simulink model "PhysicalLeanBroth"  (R2026a)
settings: Solver=VariableStepAuto  StopTime=14400
undefined symbols (not defined in the file): Fault_T_Kettle1, Fault_T_Kettle2, Fault_T_Pack, Fault_T_Prep, Fault_T_QC, LB_PackRate_bph, LB_QCRate_bph, LB_Resupply_bph, Recipe_Block_s, Recipe_Count, Resupply_Cutoff_T, Transport_Latency_s, Transport_Rate_bph
(part 2 of 2)

== system PhysicalLeanBroth/PlantServices/ServicesController ==
  in_directive : Inport  PortName=directive
  in_statusTransport : Inport  Port=2  PortName=statusTransport  Element=power_kW
  statusTransportHlth : Inport  Port=2  PortName=statusTransport  Element=health
  in_statusPower : Inport  Port=3  PortName=statusPower  Element=power_kW
  statusPowerHlth : Inport  Port=3  PortName=statusPower  Element=health
  BayHealth : MinMax  Inputs=2
  BayPower : Sum
  HealthPad : Constant
  MemberHealth : Mux
  bayDirective_c1 : Constant  Value=0
  bayDirective_c2 : Constant  Value=0
  bayDirective_c3 : Constant
  bayStatus_c1 : Constant
  bayStatus_c2 : Constant
  bayStatus_c3 : Constant  Value=0
  out_bayDirective : Outport  PortName=bayDirective  Element=cmdType
  bayDirective_el2 : Outport  PortName=bayDirective  Element=targetId
  bayDirective_el3 : Outport  PortName=bayDirective  Element=setpoint
  out_bayStatus : Outport  Port=2  PortName=bayStatus  Element=unitId
  bayStatus_el2 : Outport  Port=2  PortName=bayStatus  Element=opState
  bayStatus_el3 : Outport  Port=2  PortName=bayStatus  Element=faultCode
  bayStatus_el4 : Outport  Port=2  PortName=bayStatus  Element=power_kW
  bayStatus_el5 : Outport  Port=2  PortName=bayStatus  Element=health
  bayStatus_el6 : Outport  Port=2  PortName=bayStatus  Element=lineHealth
  wires:
  BayHealth/1 -> bayStatus_el5/1
  bayStatus_c2/1 -> bayStatus_el2/1
  bayDirective_c3/1 -> bayDirective_el3/1
  statusPowerHlth/1 -> MemberHealth/1, BayHealth/1
  bayStatus_c1/1 -> out_bayStatus/1
  bayDirective_c1/1 -> out_bayDirective/1
  bayStatus_c3/1 -> bayStatus_el3/1
  in_statusTransport/1 -> BayPower/2
  in_statusPower/1 -> BayPower/1
  HealthPad/1 -> MemberHealth/3, MemberHealth/4
  statusTransportHlth/1 -> BayHealth/2, MemberHealth/2
  bayDirective_c2/1 -> bayDirective_el2/1
  BayPower/1 -> bayStatus_el4/1
  MemberHealth/1 -> bayStatus_el6/1

== system PhysicalLeanBroth/ProductionLine/BatchKettle1 ==
  in_preppedBatch : Inport  PortName=preppedBatch  Element=flow_bps
  in_directive : Inport  Port=2  PortName=directive  Element=setpoint
  En_Gate_Fault_T_Kettle1 : Product
  Gate_Fault_T_Kettle1 : Step  Time=Fault_T_Kettle1  InitialValue=1  FinalValue=0  SampleTime=0
  HalfShare : Gain  Gain=0.5
  StateDbl : DataTypeConversion  OutDataTypeStr=double  SaturateOnIntegerOverflow=off  RndMeth=Floor
  ToLitres : Gain  Gain=1800
  Trm22 : Terminator
  Vat : ModelReference  ModelNameDialog=BehCookVat  UsingDefaultArgumentValue=0,0,0,0,0,0,0,0  SimulationMode=Normal  ModelReferenceVersion=1.9
  cookedSoup1_c1 : Constant  Value=0
  cookedSoup1_c2 : Constant  Value=0
  statusCook1_c1 : Constant
  statusCook1_c2 : Constant  Value=0
  out_cookedSoup1 : Outport  PortName=cookedSoup1  Element=batchId
  cookedSoup1_el2 : Outport  PortName=cookedSoup1  Element=volume_L
  cookedSoup1_el3 : Outport  PortName=cookedSoup1  Element=temp_C
  cookedSoup1_el4 : Outport  PortName=cookedSoup1  Element=contamination_ppm
  cookedSoup1_el5 : Outport  PortName=cookedSoup1  Element=flow_bps
  out_statusCook1 : Outport  Port=2  PortName=statusCook1  Element=unitId
  statusCook1_el2 : Outport  Port=2  PortName=statusCook1  Element=opState
  statusCook1_el3 : Outport  Port=2  PortName=statusCook1  Element=faultCode
  statusCook1_el4 : Outport  Port=2  PortName=statusCook1  Element=power_kW
  statusCook1_el5 : Outport  Port=2  PortName=statusCook1  Element=health
  wires:
  statusCook1_c2/1 -> statusCook1_el3/1
  cookedSoup1_c2/1 -> cookedSoup1_el4/1
  in_preppedBatch/1 -> HalfShare/1
  Gate_Fault_T_Kettle1/1 -> statusCook1_el5/1, En_Gate_Fault_T_Kettle1/2
  ToLitres/1 -> cookedSoup1_el2/1
  Vat/3 -> cookedSoup1_el3/1
  statusCook1_c1/1 -> out_statusCook1/1
  Vat/1 -> cookedSoup1_el5/1, ToLitres/1
  in_directive/1 -> En_Gate_Fault_T_Kettle1/1
  cookedSoup1_c1/1 -> out_cookedSoup1/1
  HalfShare/1 -> Vat/1
  En_Gate_Fault_T_Kettle1/1 -> Vat/2
  Vat/2 -> statusCook1_el4/1
  Vat/4 -> StateDbl/1
  Vat/5 -> Trm22/1
  StateDbl/1 -> statusCook1_el2/1

== system PhysicalLeanBroth/ProductionLine/BatchKettle2 ==
  in_preppedBatch : Inport  PortName=preppedBatch  Element=flow_bps
  in_directive : Inport  Port=2  PortName=directive  Element=setpoint
  En_Gate_Fault_T_Kettle2 : Product
  Gate_Fault_T_Kettle2 : Step  Time=Fault_T_Kettle2  InitialValue=1  FinalValue=0  SampleTime=0
  HalfShare : Gain  Gain=0.5
  StateDbl : DataTypeConversion  OutDataTypeStr=double  SaturateOnIntegerOverflow=off  RndMeth=Floor
  ToLitres : Gain  Gain=1800
  Trm23 : Terminator
  Vat : ModelReference  ModelNameDialog=BehCookVat  UsingDefaultArgumentValue=0,0,0,0,0,0,0,0  SimulationMode=Normal  ModelReferenceVersion=1.9
  cookedSoup2_c1 : Constant  Value=0
  cookedSoup2_c2 : Constant  Value=0
  statusCook2_c1 : Constant  Value=2
  statusCook2_c2 : Constant  Value=0
  out_cookedSoup2 : Outport  PortName=cookedSoup2  Element=batchId
  cookedSoup2_el2 : Outport  PortName=cookedSoup2  Element=volume_L
  cookedSoup2_el3 : Outport  PortName=cookedSoup2  Element=temp_C
  cookedSoup2_el4 : Outport  PortName=cookedSoup2  Element=contamination_ppm
  cookedSoup2_el5 : Outport  PortName=cookedSoup2  Element=flow_bps
  out_statusCook2 : Outport  Port=2  PortName=statusCook2  Element=unitId
  statusCook2_el2 : Outport  Port=2  PortName=statusCook2  Element=opState
  statusCook2_el3 : Outport  Port=2  PortName=statusCook2  Element=faultCode
  statusCook2_el4 : Outport  Port=2  PortName=statusCook2  Element=power_kW
  statusCook2_el5 : Outport  Port=2  PortName=statusCook2  Element=health
  wires:
  statusCook2_c2/1 -> statusCook2_el3/1
  cookedSoup2_c2/1 -> cookedSoup2_el4/1
  Gate_Fault_T_Kettle2/1 -> En_Gate_Fault_T_Kettle2/2, statusCook2_el5/1
  in_preppedBatch/1 -> HalfShare/1
  ToLitres/1 -> cookedSoup2_el2/1
  Vat/3 -> cookedSoup2_el3/1
  statusCook2_c1/1 -> out_statusCook2/1
  Vat/1 -> cookedSoup2_el5/1, ToLitres/1
  in_directive/1 -> En_Gate_Fault_T_Kettle2/1
  cookedSoup2_c1/1 -> out_cookedSoup2/1
  HalfShare/1 -> Vat/1
  En_Gate_Fault_T_Kettle2/1 -> Vat/2
  Vat/2 -> statusCook2_el4/1
  Vat/4 -> StateDbl/1
  Vat/5 -> Trm23/1
  StateDbl/1 -> statusCook2_el2/1

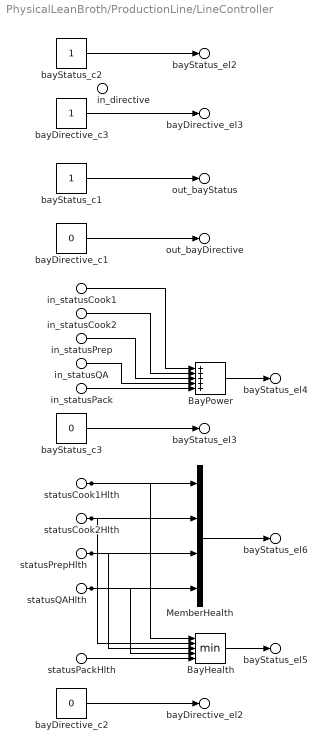
== system PhysicalLeanBroth/ProductionLine/LineController ==
  in_directive : Inport  PortName=directive
  in_statusCook1 : Inport  Port=2  PortName=statusCook1  Element=power_kW
  statusCook1Hlth : Inport  Port=2  PortName=statusCook1  Element=health
  in_statusCook2 : Inport  Port=3  PortName=statusCook2  Element=power_kW
  statusCook2Hlth : Inport  Port=3  PortName=statusCook2  Element=health
  in_statusPrep : Inport  Port=4  PortName=statusPrep  Element=power_kW
  statusPrepHlth : Inport  Port=4  PortName=statusPrep  Element=health
  in_statusQA : Inport  Port=5  PortName=statusQA  Element=power_kW
  statusQAHlth : Inport  Port=5  PortName=statusQA  Element=health
  in_statusPack : Inport  Port=6  PortName=statusPack  Element=power_kW
  statusPackHlth : Inport  Port=6  PortName=statusPack  Element=health
  BayHealth : MinMax  Inputs=5
  BayPower : Sum  Inputs=+++++
  MemberHealth : Mux
  bayDirective_c1 : Constant  Value=0
  bayDirective_c2 : Constant  Value=0
  bayDirective_c3 : Constant
  bayStatus_c1 : Constant
  bayStatus_c2 : Constant
  bayStatus_c3 : Constant  Value=0
  out_bayDirective : Outport  PortName=bayDirective  Element=cmdType
  bayDirective_el2 : Outport  PortName=bayDirective  Element=targetId
  bayDirective_el3 : Outport  PortName=bayDirective  Element=setpoint
  out_bayStatus : Outport  Port=2  PortName=bayStatus  Element=unitId
  bayStatus_el2 : Outport  Port=2  PortName=bayStatus  Element=opState
  bayStatus_el3 : Outport  Port=2  PortName=bayStatus  Element=faultCode
  bayStatus_el4 : Outport  Port=2  PortName=bayStatus  Element=power_kW
  bayStatus_el5 : Outport  Port=2  PortName=bayStatus  Element=health
  bayStatus_el6 : Outport  Port=2  PortName=bayStatus  Element=lineHealth
  wires:
  bayStatus_c2/1 -> bayStatus_el2/1
  bayStatus_c1/1 -> out_bayStatus/1
  bayDirective_c3/1 -> bayDirective_el3/1
  bayDirective_c1/1 -> out_bayDirective/1
  in_statusQA/1 -> BayPower/4
  in_statusPrep/1 -> BayPower/3
  in_statusCook2/1 -> BayPower/2
  in_statusCook1/1 -> BayPower/1
  in_statusPack/1 -> BayPower/5
  bayStatus_c3/1 -> bayStatus_el3/1
  statusCook1Hlth/1 -> BayHealth/1, MemberHealth/1
  statusCook2Hlth/1 -> BayHealth/2, MemberHealth/2
  statusPrepHlth/1 -> BayHealth/3, MemberHealth/3
  statusQAHlth/1 -> BayHealth/4, MemberHealth/4
  statusPackHlth/1 -> BayHealth/5
  bayDirective_c2/1 -> bayDirective_el2/1
  BayPower/1 -> bayStatus_el4/1
  BayHealth/1 -> bayStatus_el5/1
  MemberHealth/1 -> bayStatus_el6/1

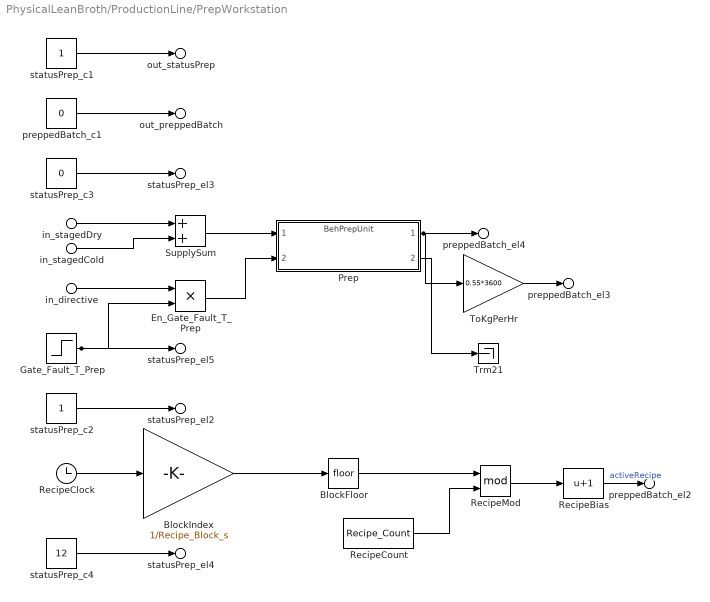
== system PhysicalLeanBroth/ProductionLine/PrepWorkstation ==
  in_stagedCold : Inport  PortName=stagedCold  Element=flow_bps
  in_stagedDry : Inport  Port=2  PortName=stagedDry  Element=flow_bps
  in_directive : Inport  Port=3  PortName=directive  Element=setpoint
  BlockFloor : Rounding
  BlockIndex : Gain  Gain=1/Recipe_Block_s
  En_Gate_Fault_T_Prep : Product
  Gate_Fault_T_Prep : Step  Time=Fault_T_Prep  InitialValue=1  FinalValue=0  SampleTime=0
  Prep : ModelReference  ModelNameDialog=BehPrepUnit  UsingDefaultArgumentValue=0,0  SimulationMode=Normal  ModelReferenceVersion=1.5
  RecipeBias : Bias  Bias=1  SaturateOnIntegerOverflow=off
  RecipeClock : Clock
  RecipeCount : Constant  Value=Recipe_Count
  RecipeMod : Math  Operator=mod
  SupplySum : Sum
  ToKgPerHr : Gain  Gain=0.55*3600
  Trm21 : Terminator
  preppedBatch_c1 : Constant  Value=0
  statusPrep_c1 : Constant
  statusPrep_c2 : Constant
  statusPrep_c3 : Constant  Value=0
  statusPrep_c4 : Constant  Value=12
  out_preppedBatch : Outport  PortName=preppedBatch  Element=batchId
  preppedBatch_el2 : Outport  PortName=preppedBatch  Element=recipeId
  preppedBatch_el3 : Outport  PortName=preppedBatch  Element=mass_kg
  preppedBatch_el4 : Outport  PortName=preppedBatch  Element=flow_bps
  out_statusPrep : Outport  Port=2  PortName=statusPrep  Element=unitId
  statusPrep_el2 : Outport  Port=2  PortName=statusPrep  Element=opState
  statusPrep_el3 : Outport  Port=2  PortName=statusPrep  Element=faultCode
  statusPrep_el4 : Outport  Port=2  PortName=statusPrep  Element=power_kW
  statusPrep_el5 : Outport  Port=2  PortName=statusPrep  Element=health
  wires:
  BlockFloor/1 -> RecipeMod/1
  in_stagedDry/1 -> SupplySum/1
  statusPrep_c1/1 -> out_statusPrep/1
  statusPrep_c3/1 -> statusPrep_el3/1
  preppedBatch_c1/1 -> out_preppedBatch/1
  Gate_Fault_T_Prep/1 -> statusPrep_el5/1, En_Gate_Fault_T_Prep/2
  in_directive/1 -> En_Gate_Fault_T_Prep/1
  in_stagedCold/1 -> SupplySum/2
  statusPrep_c2/1 -> statusPrep_el2/1
  RecipeClock/1 -> BlockIndex/1
  statusPrep_c4/1 -> statusPrep_el4/1
  SupplySum/1 -> Prep/1
  En_Gate_Fault_T_Prep/1 -> Prep/2
  BlockIndex/1 -> BlockFloor/1
  Prep/1 -> preppedBatch_el4/1, ToKgPerHr/1
  Prep/2 -> Trm21/1
  RecipeCount/1 -> RecipeMod/2
  ToKgPerHr/1 -> preppedBatch_el3/1
  RecipeMod/1 -> RecipeBias/1
  RecipeBias/1 -> preppedBatch_el2/1  "activeRecipe"

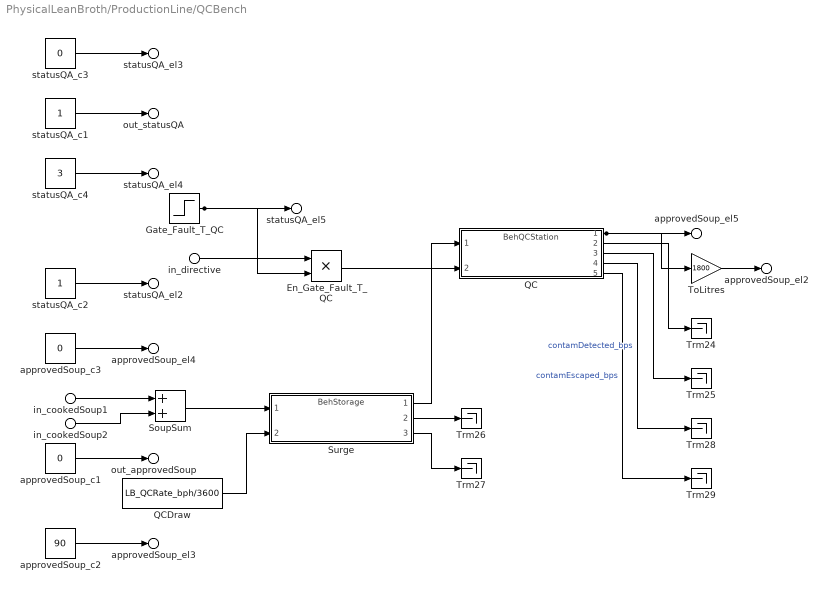
== system PhysicalLeanBroth/ProductionLine/QCBench ==
  in_cookedSoup1 : Inport  PortName=cookedSoup1  Element=flow_bps
  in_cookedSoup2 : Inport  Port=2  PortName=cookedSoup2  Element=flow_bps
  in_directive : Inport  Port=3  PortName=directive  Element=setpoint
  En_Gate_Fault_T_QC : Product
  Gate_Fault_T_QC : Step  Time=Fault_T_QC  InitialValue=1  FinalValue=0  SampleTime=0
  QC : ModelReference  ModelNameDialog=BehQCStation  UsingDefaultArgumentValue=0,0,0,0,0,0  SimulationMode=Normal  ModelReferenceVersion=1.6
  QCDraw : Constant  Value=LB_QCRate_bph/3600
  SoupSum : Sum
  Surge : ModelReference  ModelNameDialog=BehStorage  UsingDefaultArgumentValue=0,0  SimulationMode=Normal  ModelReferenceVersion=1.4
  ToLitres : Gain  Gain=1800
  Trm{24..29} (6 alike) : Terminator
  approvedSoup_c1 : Constant  Value=0
  approvedSoup_c2 : Constant  Value=90
  approvedSoup_c3 : Constant  Value=0
  statusQA_c1 : Constant
  statusQA_c2 : Constant
  statusQA_c3 : Constant  Value=0
  statusQA_c4 : Constant  Value=3
  out_approvedSoup : Outport  PortName=approvedSoup  Element=batchId
  approvedSoup_el2 : Outport  PortName=approvedSoup  Element=volume_L
  approvedSoup_el3 : Outport  PortName=approvedSoup  Element=temp_C
  approvedSoup_el4 : Outport  PortName=approvedSoup  Element=contamination_ppm
  approvedSoup_el5 : Outport  PortName=approvedSoup  Element=flow_bps
  out_statusQA : Outport  Port=2  PortName=statusQA  Element=unitId
  statusQA_el2 : Outport  Port=2  PortName=statusQA  Element=opState
  statusQA_el3 : Outport  Port=2  PortName=statusQA  Element=faultCode
  statusQA_el4 : Outport  Port=2  PortName=statusQA  Element=power_kW
  statusQA_el5 : Outport  Port=2  PortName=statusQA  Element=health
  wires:
  in_cookedSoup2/1 -> SoupSum/2
  statusQA_c3/1 -> statusQA_el3/1
  statusQA_c1/1 -> out_statusQA/1
  statusQA_c4/1 -> statusQA_el4/1
  Surge/2 -> Trm26/1
  statusQA_c2/1 -> statusQA_el2/1
  approvedSoup_c3/1 -> approvedSoup_el4/1
  approvedSoup_c1/1 -> out_approvedSoup/1
  in_cookedSoup1/1 -> SoupSum/1
  approvedSoup_c2/1 -> approvedSoup_el3/1
  Gate_Fault_T_QC/1 -> statusQA_el5/1, En_Gate_Fault_T_QC/2
  in_directive/1 -> En_Gate_Fault_T_QC/1
  Surge/3 -> Trm27/1
  SoupSum/1 -> Surge/1
  QCDraw/1 -> Surge/2
  En_Gate_Fault_T_QC/1 -> QC/2
  Surge/1 -> QC/1
  QC/1 -> approvedSoup_el5/1, ToLitres/1
  QC/2 -> Trm24/1
  QC/3 -> Trm25/1
  QC/4 -> Trm28/1  "contamDetected_bps"
  QC/5 -> Trm29/1  "contamEscaped_bps"
  ToLitres/1 -> approvedSoup_el2/1

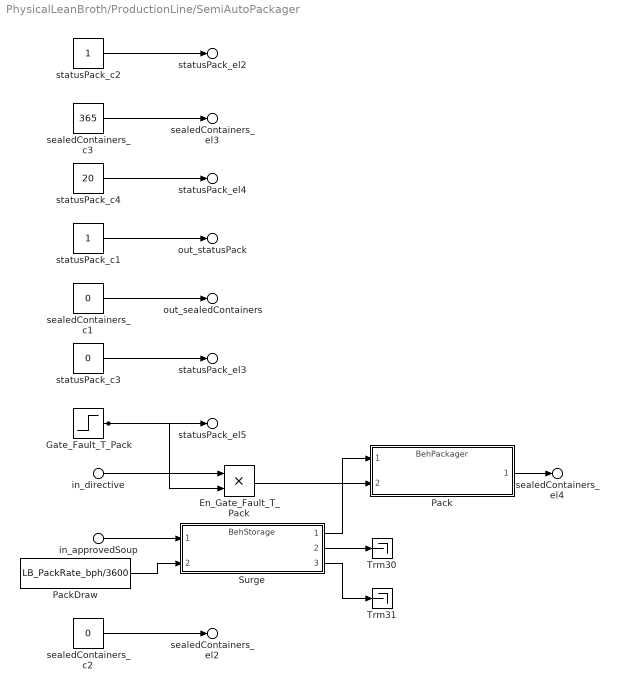
== system PhysicalLeanBroth/ProductionLine/SemiAutoPackager ==
  in_approvedSoup : Inport  PortName=approvedSoup  Element=flow_bps
  in_directive : Inport  Port=2  PortName=directive  Element=setpoint
  En_Gate_Fault_T_Pack : Product
  Gate_Fault_T_Pack : Step  Time=Fault_T_Pack  InitialValue=1  FinalValue=0  SampleTime=0
  Pack : ModelReference  ModelNameDialog=BehPackager  UsingDefaultArgumentValue=0,0  SimulationMode=Normal  ModelReferenceVersion=1.5
  PackDraw : Constant  Value=LB_PackRate_bph/3600
  Surge : ModelReference  ModelNameDialog=BehStorage  UsingDefaultArgumentValue=0,0  SimulationMode=Normal  ModelReferenceVersion=1.4
  Trm30 : Terminator
  Trm31 : Terminator
  sealedContainers_c1 : Constant  Value=0
  sealedContainers_c2 : Constant  Value=0
  sealedContainers_c3 : Constant  Value=365
  statusPack_c1 : Constant
  statusPack_c2 : Constant
  statusPack_c3 : Constant  Value=0
  statusPack_c4 : Constant  Value=20
  out_sealedContainers : Outport  PortName=sealedContainers  Element=batchId
  sealedContainers_el2 : Outport  PortName=sealedContainers  Element=count
  sealedContainers_el3 : Outport  PortName=sealedContainers  Element=sealRating_days
  sealedContainers_el4 : Outport  PortName=sealedContainers  Element=flow_bps
  out_statusPack : Outport  Port=2  PortName=statusPack  Element=unitId
  statusPack_el2 : Outport  Port=2  PortName=statusPack  Element=opState
  statusPack_el3 : Outport  Port=2  PortName=statusPack  Element=faultCode
  statusPack_el4 : Outport  Port=2  PortName=statusPack  Element=power_kW
  statusPack_el5 : Outport  Port=2  PortName=statusPack  Element=health
  wires:
  statusPack_c2/1 -> statusPack_el2/1
  En_Gate_Fault_T_Pack/1 -> Pack/2
  in_directive/1 -> En_Gate_Fault_T_Pack/1
  sealedContainers_c1/1 -> out_sealedContainers/1
  sealedContainers_c3/1 -> sealedContainers_el3/1
  statusPack_c4/1 -> statusPack_el4/1
  statusPack_c1/1 -> out_statusPack/1
  Gate_Fault_T_Pack/1 -> En_Gate_Fault_T_Pack/2, statusPack_el5/1
  Surge/1 -> Pack/1
  statusPack_c3/1 -> statusPack_el3/1
  in_approvedSoup/1 -> Surge/1
  PackDraw/1 -> Surge/2
  sealedContainers_c2/1 -> sealedContainers_el2/1
  Surge/2 -> Trm30/1
  Surge/3 -> Trm31/1
  Pack/1 -> sealedContainers_el4/1
